simulink model "NeedleMotion"  (Simulink 7.7)
settings: Solver=FixedStepDiscrete  StartTime=0.0  StopTime=tf  FixedStep=dt  MaxStep=dt  RelTol=1e-3
values from neighbouring files (symbols this model uses):
  dt = 0.0001    [SimpleNeedleMotion.m]
  P0 = zeros(7,1)    [SimpleNeedleMotion.m]
  Vel = randn(6,1)    [SimpleNeedleMotion.m]
settings Model: Creator=mercislab  LastModifiedBy=rcj33
settings DebuggingCC: FcnCallInpInsideContextMsg=Enable All

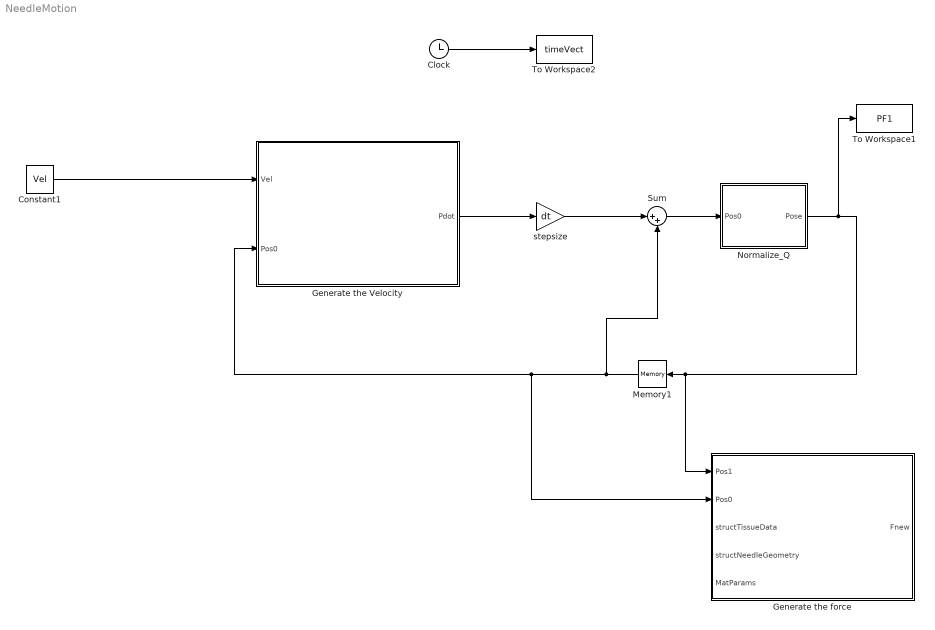
== system NeedleMotion ==
  Clock : Clock
      settings: Decimation=10
  Constant1 : Constant  Value=Vel
  Generate the Velocity : Stateflow chart  TreatAsAtomicUnit=on
  Generate the force : Stateflow chart  TreatAsAtomicUnit=on
  Memory1 : Memory  X0=P0
  Normalize_Q : Stateflow chart  TreatAsAtomicUnit=on
  Sum : Sum  Inputs=|++
  To Workspace1 : ToWorkspace  VariableName=PF1  SampleTime=-1  SaveFormat=Structure
  To Workspace2 : ToWorkspace  VariableName=timeVect  SampleTime=-1  SaveFormat=Structure
  stepsize : Gain  Gain=dt
  wires:
  Memory1/1 -> Sum/2, Generate the Velocity/2(Pos0), Generate the force/2(Pos0)
  Generate the Velocity/1(Pdot) -> stepsize/1
  stepsize/1 -> Sum/1
  Sum/1 -> Normalize_Q/1(Pos0)
  Normalize_Q/1(Pose) -> To Workspace1/1, Memory1/1, Generate the force/1(Pos1)
  Constant1/1 -> Generate the Velocity/1(Vel)
  Clock/1 -> To Workspace2/1

== matlab function Generate the Velocity ==
  data: Vel input double; Pos0 input double; Pdot output double
function Pdot = PoseV(Vel,Pos0)
  %Note the body is in the body frame so rotate the translational velocity.
  

    
  %#codegen
  q0 = Pos0(4:7);
  W  = [0; Vel(4:6)];
  
  PdotQ = 0.5*QaXQb(W,q0)';
  
  r0 = Q2R(q0);

  PdotV =  r0*Vel(1:3);
  
  Pdot = [PdotV; PdotQ];
  
  
  
  
end

== matlab function Normalize_Q ==
  data: Pos0 input double; Pose output double
function Pose = Renormal(Pos0)
  %Note the body is in the body frame so rotate the translational velocity.
  

    
  %#codegen
  PoseQ = Pos0(4:7);
  
  NQ = norm(PoseQ);
  
  PoseQ = PoseQ/NQ;
  
  Pose = [Pos0(1:3); PoseQ];
  
  
  
  
end

== matlab function Generate the force ==
  data: Pos1 input double; Pos0 input double; Fnew output double; structTissueData input double; structNeedleGeometry input double; MatParams input double
function Fnew = Force(Pos1,Pos0,structTissueData,structNeedleGeometry,MatParams)
 %This function generates the forces on the Needle and how they change as a
 %function of position
 %#codegen
 
 
 [TissueState  NeedlePts2]=Needle_Tissue_Intersection(structTissueData,structNeedleGeometry,NeedleTransDes,100);Needle_Tissue_Intersection(structTissueData,structNeedleGeometry,NeedleTransDes,100);

    
  
  q0 = Pos0(4:7);
  W  = [0; Vel(4:6)];
  
  PdotQ = 0.5*QaXQb(W,q0)';
  
  r0 = Q2R(q0);

  PdotV =  r0*Vel(1:3);
  
  Pdot = [PdotV; PdotQ];
  
  
  
  
end
